simulink model "GPCA_Top_Level_Mode_2015a"  (Simulink 8.5)
settings: Solver=ode45  StartTime=0.0  StopTime=10.0  RelTol=1e-3
settings Model: Creator=bourbouh  LastModifiedBy=hamza  CovModelRefEnable=off
settings DataIOCC: LimitDataPoints=off  SaveFormat=Dataset  SignalLoggingSaveFormat=Dataset
settings OptimizationCC: ExpressionDepthLimit=128
settings DebuggingCC: UnderspecifiedInitializationDetection=Simplified  MergeDetectMultiDrivingBlocksExec=error  FcnCallInpInsideContextMsg=EnableAllAsError  StateNameClashWarn=none
settings HardwareCC: ProdBitPerPointer=64  ProdLargestAtomicFloat=Float  ProdIntDivRoundTo=Zero  ProdEndianess=LittleEndian  ProdHWDeviceType=Specified
settings ModelReferenceCC: PropagateSignalLabelsOutOfModel=on
settings GRTTargetCC: CombineOutputUpdateFcns=on  GRTInterface=off

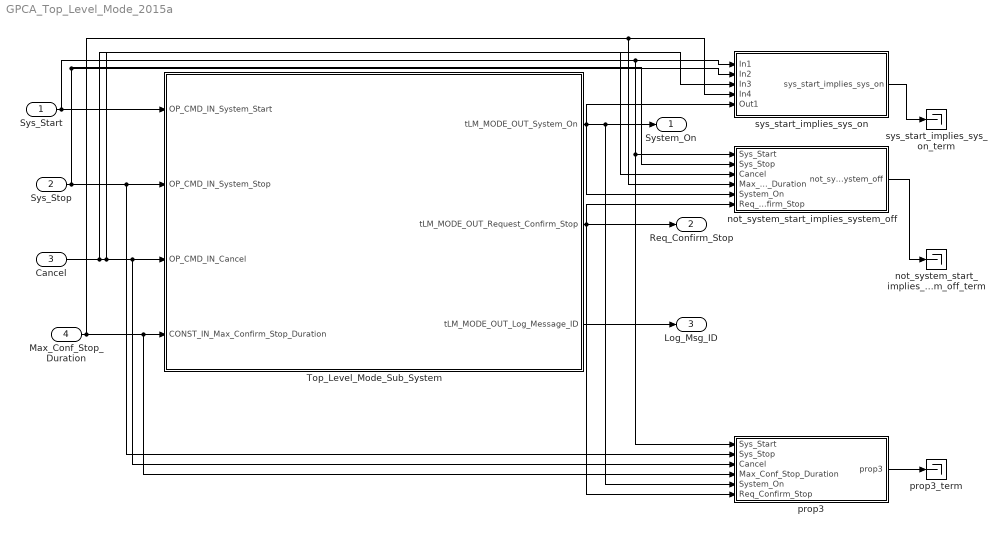
== system GPCA_Top_Level_Mode_2015a ==
  Sys_Start : Inport
  Sys_Stop : Inport  Port=2
  Cancel : Inport  Port=3
  Max_Conf_Stop_Duration : Inport  Port=4
  Top_Level_Mode_Sub_System : Stateflow chart  TreatAsAtomicUnit=on
      settings: PermitHierarchicalResolution=ParametersOnly
  not_system_start_implies_system_off : Subsystem  TreatAsAtomicUnit=on  mask(Observer){AnnotationType=ensures, ObserverType=[]}
      mask prompts: AnnotationType "Type of annotation (pre/post...)"; ObserverType "Observer type"
      mask help:
      | Set an observer for the system.
      | The annotation type parameter sets the type of observer:
      | - requires : pre-condition
      | - ensures : post-condition
      | - assert : an assertion
      | - observer : the observer computes a special type of properties
      mask TypeOptions AnnotationType: ensures | requires | assert | observer
      mask Callback AnnotationType:
      | paramStr = get_param(gcb, 'MaskValues');
      | if strcmp(paramStr{1}(1),'o')
      | set_param(gcb,'MaskVisibilities',{'on';'on'});
      | paramStr{2} = 'ellipsoid';
      | set_param(gcb,'MaskValues',paramStr);
      | else
      | set_param(gcb,'MaskVisibilities',{'on';'off'});
      | end
      | clear paramStr;
      mask Callback ObserverType:
      | paramStr = get_param(gcb, 'MaskValues');
      | if strcmp(paramStr{1}(1),'o')
      | set_param(gcb,'MaskVisibilities',{'on';'on'});
      | paramStr{2} = 'ellipsoid';
      | set_param(gcb,'MaskValues',paramStr);
      | else
      | set_param(gcb,'MaskVisibilities',{'on';'off'});
      | end
      | clear paramStr;
      mask Display:
      | color('black')
      | text(0.5, 0.5, ['Property: ''' get_param(gcb,'name') ''''], 'horizontalAlignment', 'center');
      | text(0.99, 0.03, '{\bf\fontsize{12}SAFE}', 'hor', 'right', 'ver', 'bottom', 'texmode', 'on');
  not_system_start_implies_system_off_term : Terminator
  prop3 : Subsystem  TreatAsAtomicUnit=on  mask(Observer){AnnotationType=ensures, ObserverType=[]}
      mask prompts: AnnotationType "Type of annotation (pre/post...)"; ObserverType "Observer type"
      mask help:
      | Set an observer for the system.
      | The annotation type parameter sets the type of observer:
      | - requires : pre-condition
      | - ensures : post-condition
      | - assert : an assertion
      | - observer : the observer computes a special type of properties
      mask TypeOptions AnnotationType: ensures | requires | assert | observer
      mask Callback AnnotationType:
      | paramStr = get_param(gcb, 'MaskValues');
      | if strcmp(paramStr{1}(1),'o')
      | set_param(gcb,'MaskVisibilities',{'on';'on'});
      | paramStr{2} = 'ellipsoid';
      | set_param(gcb,'MaskValues',paramStr);
      | else
      | set_param(gcb,'MaskVisibilities',{'on';'off'});
      | end
      | clear paramStr;
      mask Callback ObserverType:
      | paramStr = get_param(gcb, 'MaskValues');
      | if strcmp(paramStr{1}(1),'o')
      | set_param(gcb,'MaskVisibilities',{'on';'on'});
      | paramStr{2} = 'ellipsoid';
      | set_param(gcb,'MaskValues',paramStr);
      | else
      | set_param(gcb,'MaskVisibilities',{'on';'off'});
      | end
      | clear paramStr;
      mask Display:
      | color('black')
      | text(0.5, 0.5, ['Property: ''' get_param(gcb,'name') ''''], 'horizontalAlignment', 'center');
      | text(0.99, 0.03, '{\bf\fontsize{12}SAFE}', 'hor', 'right', 'ver', 'bottom', 'texmode', 'on');
  prop3_term : Terminator
  sys_start_implies_sys_on : Subsystem  TreatAsAtomicUnit=on  mask(Observer){AnnotationType=ensures, ObserverType=[]}
      mask prompts: AnnotationType "Type of annotation (pre/post...)"; ObserverType "Observer type"
      mask help:
      | Set an observer for the system.
      | The annotation type parameter sets the type of observer:
      | - requires : pre-condition
      | - ensures : post-condition
      | - assert : an assertion
      | - observer : the observer computes a special type of properties
      mask TypeOptions AnnotationType: ensures | requires | assert | observer
      mask Callback AnnotationType:
      | paramStr = get_param(gcb, 'MaskValues');
      | if strcmp(paramStr{1}(1),'o')
      | set_param(gcb,'MaskVisibilities',{'on';'on'});
      | paramStr{2} = 'ellipsoid';
      | set_param(gcb,'MaskValues',paramStr);
      | else
      | set_param(gcb,'MaskVisibilities',{'on';'off'});
      | end
      | clear paramStr;
      mask Callback ObserverType:
      | paramStr = get_param(gcb, 'MaskValues');
      | if strcmp(paramStr{1}(1),'o')
      | set_param(gcb,'MaskVisibilities',{'on';'on'});
      | paramStr{2} = 'ellipsoid';
      | set_param(gcb,'MaskValues',paramStr);
      | else
      | set_param(gcb,'MaskVisibilities',{'on';'off'});
      | end
      | clear paramStr;
      mask Display:
      | color('black')
      | text(0.5, 0.5, ['Property: ''' get_param(gcb,'name') ''''], 'horizontalAlignment', 'center');
      | text(0.99, 0.03, '{\bf\fontsize{12}SAFE}', 'hor', 'right', 'ver', 'bottom', 'texmode', 'on');
  sys_start_implies_sys_on_term : Terminator
  System_On : Outport
  Req_Confirm_Stop : Outport  Port=2
  Log_Msg_ID : Outport  Port=3
  wires:
  Sys_Start/1 -> not_system_start_implies_system_off/1(Sys_Start), prop3/1(Sys_Start), sys_start_implies_sys_on/1(In1), Top_Level_Mode_Sub_System/1(OP_CMD_IN_System_Start)
  Sys_Stop/1 -> sys_start_implies_sys_on/2(In2), not_system_start_implies_system_off/2(Sys_Stop), Top_Level_Mode_Sub_System/2(OP_CMD_IN_System_Stop), prop3/2(Sys_Stop)
  Cancel/1 -> sys_start_implies_sys_on/3(In3), Top_Level_Mode_Sub_System/3(OP_CMD_IN_Cancel), prop3/3(Cancel), not_system_start_implies_system_off/3(Cancel)
  Max_Conf_Stop_Duration/1 -> sys_start_implies_sys_on/4(In4), not_system_start_implies_system_off/4(Max_Conf_Stop_Duration), Top_Level_Mode_Sub_System/4(CONST_IN_Max_Confirm_Stop_Duration), prop3/4(Max_Conf_Stop_Duration)
  Top_Level_Mode_Sub_System/1(tLM_MODE_OUT_System_On) -> System_On/1, prop3/5(System_On), sys_start_implies_sys_on/5(Out1), not_system_start_implies_system_off/5(System_On)
  Top_Level_Mode_Sub_System/2(tLM_MODE_OUT_Request_Confirm_Stop) -> Req_Confirm_Stop/1, not_system_start_implies_system_off/6(Req_Confirm_Stop), prop3/6(Req_Confirm_Stop)
  Top_Level_Mode_Sub_System/3(tLM_MODE_OUT_Log_Message_ID) -> Log_Msg_ID/1
  sys_start_implies_sys_on/1(sys_start_implies_sys_on) -> sys_start_implies_sys_on_term/1
  not_system_start_implies_system_off/1(not_system_start_implies_system_off) -> not_system_start_implies_system_off_term/1
  prop3/1(prop3) -> prop3_term/1

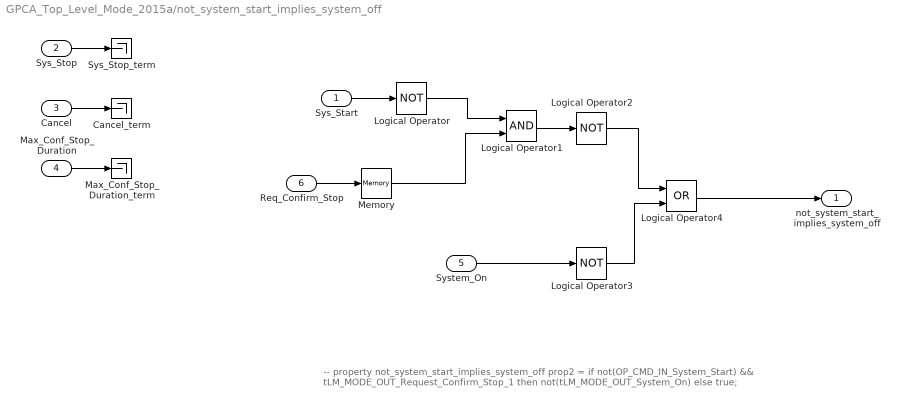
== system GPCA_Top_Level_Mode_2015a/not_system_start_implies_system_off ==
  note: -- property not_system_start_implies_system_off
      |
      | 	prop2 = if not(OP_CMD_IN_System_Start) &&  tLM_MODE_OUT_Request_Confirm_Stop_1 then not(tLM_MODE_OUT_System_On)  else true;
  Sys_Start : Inport
  Sys_Stop : Inport  Port=2
  Cancel : Inport  Port=3
  Max_Conf_Stop_Duration : Inport  Port=4
  System_On : Inport  Port=5
  Req_Confirm_Stop : Inport  Port=6
  Cancel_term : Terminator
  Logical Operator : Logic  Operator=NOT  AllPortsSameDT=off  OutDataTypeStr=boolean
  Logical Operator1 : Logic  AllPortsSameDT=off  OutDataTypeStr=boolean
  Logical Operator2 : Logic  Operator=NOT  AllPortsSameDT=off  OutDataTypeStr=boolean
  Logical Operator3 : Logic  Operator=NOT  AllPortsSameDT=off  OutDataTypeStr=boolean
  Logical Operator4 : Logic  Operator=OR  AllPortsSameDT=off  OutDataTypeStr=boolean
  Max_Conf_Stop_Duration_term : Terminator
  Memory : Memory
  Sys_Stop_term : Terminator
  not_system_start_implies_system_off : Outport
  wires:
  Sys_Start/1 -> Logical Operator/1
  Sys_Stop/1 -> Sys_Stop_term/1
  Cancel/1 -> Cancel_term/1
  Max_Conf_Stop_Duration/1 -> Max_Conf_Stop_Duration_term/1
  System_On/1 -> Logical Operator3/1
  Req_Confirm_Stop/1 -> Memory/1
  Memory/1 -> Logical Operator1/2
  Logical Operator/1 -> Logical Operator1/1
  Logical Operator1/1 -> Logical Operator2/1
  Logical Operator2/1 -> Logical Operator4/1
  Logical Operator3/1 -> Logical Operator4/2
  Logical Operator4/1 -> not_system_start_implies_system_off/1

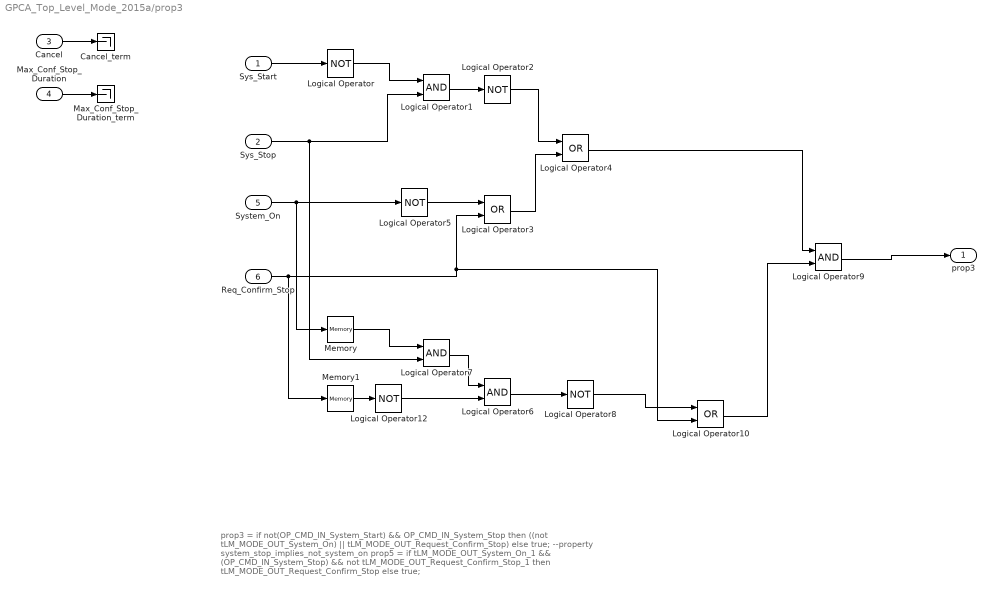
== system GPCA_Top_Level_Mode_2015a/prop3 ==
  note: prop3 = if not(OP_CMD_IN_System_Start) &&  OP_CMD_IN_System_Stop  then ((not tLM_MODE_OUT_System_On) || tLM_MODE_OUT_Request_Confirm_Stop) else true;
      |
      | --property system_stop_implies_not_system_on
      | 	prop5 = if tLM_MODE_OUT_System_On_1 && (OP_CMD_IN_System_Stop) && not tLM_MODE_OUT_Request_Confirm_Stop_1  then tLM_MODE_OUT_Request_Confirm_Stop else true;
  Sys_Start : Inport
  Sys_Stop : Inport  Port=2
  Cancel : Inport  Port=3
  Max_Conf_Stop_Duration : Inport  Port=4
  System_On : Inport  Port=5
  Req_Confirm_Stop : Inport  Port=6
  Cancel_term : Terminator
  Logical Operator{,2,5,8,12} (5 alike) : Logic  Operator=NOT  AllPortsSameDT=off  OutDataTypeStr=boolean
  Logical Operator{1,6..7,9} (4 alike) : Logic  AllPortsSameDT=off  OutDataTypeStr=boolean
  Logical Operator10 : Logic  Operator=OR  AllPortsSameDT=off  OutDataTypeStr=boolean
  Logical Operator3 : Logic  Operator=OR  AllPortsSameDT=off  OutDataTypeStr=boolean
  Logical Operator4 : Logic  Operator=OR  AllPortsSameDT=off  OutDataTypeStr=boolean
  Max_Conf_Stop_Duration_term : Terminator
  Memory : Memory
  Memory1 : Memory
  prop3 : Outport
  wires:
  Cancel/1 -> Cancel_term/1
  Max_Conf_Stop_Duration/1 -> Max_Conf_Stop_Duration_term/1
  System_On/1 -> Memory/1, Logical Operator5/1
  Logical Operator/1 -> Logical Operator1/1
  Logical Operator1/1 -> Logical Operator2/1
  Logical Operator2/1 -> Logical Operator4/1
  Logical Operator3/1 -> Logical Operator4/2
  Logical Operator4/1 -> Logical Operator9/1
  Logical Operator5/1 -> Logical Operator3/1
  Sys_Start/1 -> Logical Operator/1
  Sys_Stop/1 -> Logical Operator7/2, Logical Operator1/2
  Memory/1 -> Logical Operator7/1
  Logical Operator7/1 -> Logical Operator6/1
  Logical Operator8/1 -> Logical Operator10/1
  Logical Operator10/1 -> Logical Operator9/2
  Memory1/1 -> Logical Operator12/1
  Logical Operator12/1 -> Logical Operator6/2
  Logical Operator6/1 -> Logical Operator8/1
  Req_Confirm_Stop/1 -> Logical Operator10/2, Logical Operator3/2, Memory1/1
  Logical Operator9/1 -> prop3/1

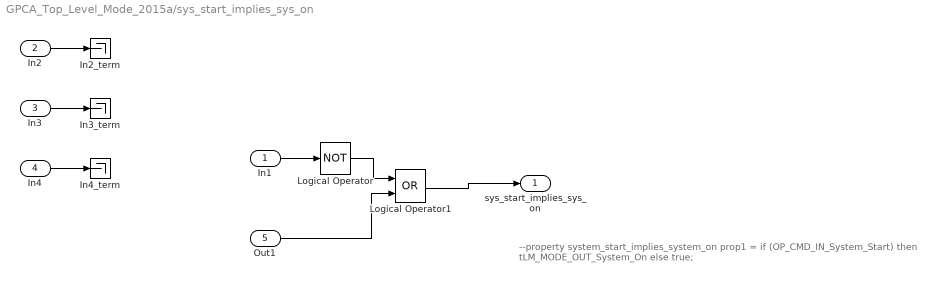
== system GPCA_Top_Level_Mode_2015a/sys_start_implies_sys_on ==
  note: --property system_start_implies_system_on
      | 	prop1 = if (OP_CMD_IN_System_Start) then  tLM_MODE_OUT_System_On else true;
  In1 : Inport
  In2 : Inport  Port=2
  In3 : Inport  Port=3
  In4 : Inport  Port=4
  Out1 : Inport  Port=5
  In2_term : Terminator
  In3_term : Terminator
  In4_term : Terminator
  Logical Operator : Logic  Operator=NOT  AllPortsSameDT=off  OutDataTypeStr=boolean
  Logical Operator1 : Logic  Operator=OR  AllPortsSameDT=off  OutDataTypeStr=boolean
  sys_start_implies_sys_on : Outport
  wires:
  In1/1 -> Logical Operator/1
  In2/1 -> In2_term/1
  In3/1 -> In3_term/1
  In4/1 -> In4_term/1
  Out1/1 -> Logical Operator1/2
  Logical Operator/1 -> Logical Operator1/1
  Logical Operator1/1 -> sys_start_implies_sys_on/1

== stateflow chart Top_Level_Mode_Sub_System ==
  state TOP_Level_Mode
    entry: tLM_MODE_OUT_System_On=1;
    during: tLM_MODE_OUT_System_On=1;
    exit: tLM_MODE_OUT_System_On=1;
    state Confirm_Stop
      state OFF
        entry:tLM_MODE_OUT_Request_Confirm_Stop=0;
        confirmStopTimer=0;
      state ON
        entry: tLM_MODE_OUT_Request_Confirm_Stop=1;
        confirmStopTimer++;
        during :confirmStopTimer++;
      (default) -> OFF [order 2]
      (default) -> ON [order 1] : [OP_CMD_IN_System_Stop]
      ON -> OFF [order 2] : [OP_CMD_IN_Cancel || confirmStopTimer > Step_Scaling_Factor(CONST_IN_Max_Confirm_Stop_Duration,step_size)]
      OFF -> ON : [OP_CMD_IN_System_Stop]
    (default) -> Confirm_Stop
  state NOT_ON
    entry: tLM_MODE_OUT_System_On=0;
    during: tLM_MODE_OUT_System_On=0;
    exit: tLM_MODE_OUT_System_On=0;
  note: The confirmation to stop the system
      | is abstracted here as !System_Start
  state returnVal = Step_Scaling_Factor(inputVal,step_size) [function]
    (default) -> (junction 20) : {returnVal=inputVal/step_size;}
  state writeLog(logEvent) [function]
    (default) -> (junction 23) : {tLM_MODE_OUT_Log_Message_ID=logEvent;}
  note: step scaling factor returns the scaled time depending upon the step size.
      | If counter has to timeout after 100 seconds and if the step size is 0.1 second
      | the new timeout value = 100/0.1 = 1000 steps.
      | default will be one step = 1 second.
  (default) -> TOP_Level_Mode [order 1] : [OP_CMD_IN_System_Start]
  (default) -> NOT_ON [order 2]
  NOT_ON -> TOP_Level_Mode : [OP_CMD_IN_System_Start]{writeLog(1);}
  ON -> NOT_ON [order 1] : [!OP_CMD_IN_System_Start]{writeLog(2);}
  data: inputVal function_input double; returnVal function_output double; step_size function_input double; logEvent function_input uint8; tLM_MODE_OUT_System_On output boolean; tLM_MODE_OUT_Request_Confirm_Stop output boolean; OP_CMD_IN_System_Start input boolean; OP_CMD_IN_System_Stop input boolean; OP_CMD_IN_Cancel input boolean; CONST_IN_Max_Confirm_Stop_Duration input double; step_size parameter double; tLM_MODE_OUT_Log_Message_ID output uint8; confirmStopTimer local double
